simulink model "motor_pendulum_system"  (R2020b)
settings: Solver=VariableStepAuto  StartTime=0.0  StopTime=1  MaxStep=1e-3  RelTol=1e-6
model workspace: external: MATLAB File /Users/sam/GitHub/3-Phase-Motor/Matlab/motor_with_new_controller.m (data not in the file)
values from neighbouring files (symbols this model uses):
  B_m = 1e-3    (= 0.001)    [Calculate_Static.m]    (also in closed_form.m; motor_with_new_controller.m)
  J = 1e-4    (= 0.0001)    [Calculate_Static.m]    (also in closed_form.m; motor_with_new_controller.m)
  K = 0.088    [Calculate_Static.m]    (also in closed_form.m; motor_with_new_controller.m)
libraries: cstblocks x2, pid_lib x2
settings Model: Creator=sam  LastModifiedBy=sam
settings ModelReferenceCC: UpdateModelReferenceTargets=Force

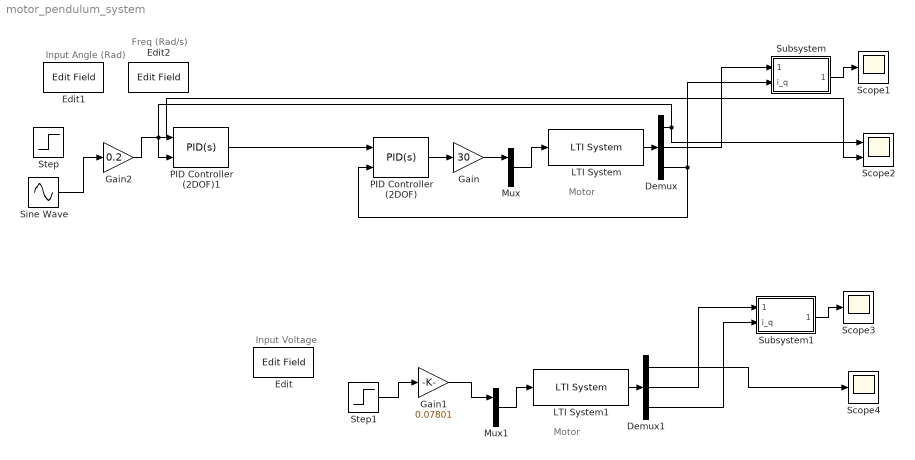
== system motor_pendulum_system ==
  note: Input Voltage
  note: Motor
  note: Motor
  note: Input Angle (Rad)
  note: Freq (Rad/s)
  Demux : Demux  Outputs=3
  Demux1 : Demux  Outputs=3
  Edit : EditField  LabelPosition=Hide  ShowInitialText=on  Alignment=Center
  Edit1 : EditField  LabelPosition=Hide  ShowInitialText=on  Alignment=Center
  Edit2 : EditField  LabelPosition=Hide  ShowInitialText=on  Alignment=Center
  Gain : Gain  Gain=30
  Gain1 : Gain  Gain=0.07801
  Gain2 : Gain  Gain=0.2
  LTI System : cstblocks/LTI System  sys=S  IC=[]
  LTI System1 : cstblocks/LTI System  sys=S  IC=[]
  Mux : Mux  Inputs=3
  Mux1 : Mux  Inputs=3
  PID Controller (2DOF) : pid_lib/PID Controller (2DOF)  Controller=PID  Form=Parallel  TimeDomain=Continuous-time  UseExternalTs=off  SampleTime=-1  IntegratorMethod=Forward Euler  FilterMethod=Forward Euler  ControllerParametersSource=internal  P=.05  I=.005  D=0  UseFilter=on  N=100  b=1  c=1  TunerSelectOption=Transfer Function Based (PID Tuner App)  InitialConditionSource=internal  InitialConditionForIntegrator=0  InitialConditionForFilter=0  DifferentiatorICPrevScaledInput=0  ExternalReset=none  TrackingMode=off  Kt=1  LimitOutput=off  SatLimitsSource=internal  UpperSaturationLimit=inf  LowerSaturationLimit=-inf  LinearizeAsGain=on  AntiWindupMode=none  Kb=1  POutMin=[]  POutMax=[]  IOutMin=[]  IOutMax=[]  DOutMin=[]  DOutMax=[]  NOutMin=[]  NOutMax=[]  bOutMin=[]  bOutMax=[]  cOutMin=[]  cOutMax=[]  SumOutMin=[]  SumOutMax=[]  SaturationOutMin=[]  SaturationOutMax=[]  PParamMin=[]  PParamMax=[]  IParamMin=[]  IParamMax=[]  DParamMin=[]  DParamMax=[]  NParamMin=[]  NParamMax=[]  bParamMin=[]  bParamMax=[]  cParamMin=[]  cParamMax=[]  KbParamMin=[]  KbParamMax=[]  KtParamMin=[]  KtParamMax=[]  KbOutMin=[]  KbOutMax=[]  KtOutMin=[]  KtOutMax=[]  IntegratorOutMin=[]  IntegratorOutMax=[]  FilterOutMin=[]  FilterOutMax=[]  SumI1OutMin=[]  SumI1OutMax=[]  SumI2OutMin=[]  SumI2OutMax=[]  SumI3OutMin=[]  SumI3OutMax=[]  SumI4OutMin=[]  SumI4OutMax=[]  SumDOutMin=[]  SumDOutMax=[]  Sum1OutMin=[]  Sum1OutMax=[]  Sum2OutMin=[]  Sum2OutMax=[]  Sum3OutMin=[]  Sum3OutMax=[]  DifferentiatorOutMin=[]  DifferentiatorOutMax=[]  FilterDiffOutCoefMin=[]  FilterDiffOutCoefMax=[]  ReciprocalOutMin=[]  ReciprocalOutMax=[]  SumDenOutMin=[]  SumDenOutMax=[]  SumNumOutMin=[]  SumNumOutMax=[]  DivideOutMin=[]  DivideOutMax=[]  UdiffTsProdOutMin=[]  UdiffTsProdOutMax=[]  NTsProdOutMin=[]  NTsProdOutMax=[]  UintegralTsProdOutMin=[]  UintegralTsProdOutMax=[]  UngainTsProdOutMin=[]  UngainTsProdOutMax=[]  IntegratorContinuousStateAttributes=''  IntegratorStateMustResolveToSignalObject=off  IntegratorRTWStateStorageClass=Auto  FilterContinuousStateAttributes=''  FilterStateMustResolveToSignalObject=off  FilterRTWStateStorageClass=Auto  ParallelPVariant=InternalParameters  IdealPVariant=Disabled  IVariant=InternalParameters  DVariant=InternalParameters  bVariant=InternalParameters  cVariant=InternalParameters  IntegratorVariant=Continuous  SatVariant=Disabled  AWVariant=Passthrough  PCopyVariant=Disabled  TRVariant=Disabled  FdbkBlocksVariant=Forward  IdealPFdbkVariant=Disabled  SatFdbkVariant=Disabled  DerivativeFilterVariant=ContFilter  NVariant=InternalParameters  NCopyVariant=Disabled  FilterICVariant=InternalICsFilter  IntegratorICVariant=InternalICs  ExternalResetVariant=Disabled  TRSumVariant=Passthrough  SumFdbkVariant=Disabled  SumVariant=Sum_PID  TsampFilterVariant=InternalTs  TsampNgainVariant=Passthrough  TsampIntegralVariant=Passthrough  ExternalSaturationOutDataTypeStr=Inherit: Same as second input
      settings: SourceProductBaseCode=SL
  PID Controller (2DOF)1 : pid_lib/PID Controller (2DOF)  Controller=PID  Form=Parallel  TimeDomain=Continuous-time  UseExternalTs=off  SampleTime=-1  IntegratorMethod=Forward Euler  FilterMethod=Forward Euler  ControllerParametersSource=internal  P=250  I=20  D=5  UseFilter=on  N=100  b=1  c=1  TunerSelectOption=Transfer Function Based (PID Tuner App)  InitialConditionSource=internal  InitialConditionForIntegrator=0  InitialConditionForFilter=0  DifferentiatorICPrevScaledInput=0  ExternalReset=none  TrackingMode=off  Kt=1  LimitOutput=off  SatLimitsSource=internal  UpperSaturationLimit=inf  LowerSaturationLimit=-inf  LinearizeAsGain=on  AntiWindupMode=none  Kb=1  POutMin=[]  POutMax=[]  IOutMin=[]  IOutMax=[]  DOutMin=[]  DOutMax=[]  NOutMin=[]  NOutMax=[]  bOutMin=[]  bOutMax=[]  cOutMin=[]  cOutMax=[]  SumOutMin=[]  SumOutMax=[]  SaturationOutMin=[]  SaturationOutMax=[]  PParamMin=[]  PParamMax=[]  IParamMin=[]  IParamMax=[]  DParamMin=[]  DParamMax=[]  NParamMin=[]  NParamMax=[]  bParamMin=[]  bParamMax=[]  cParamMin=[]  cParamMax=[]  KbParamMin=[]  KbParamMax=[]  KtParamMin=[]  KtParamMax=[]  KbOutMin=[]  KbOutMax=[]  KtOutMin=[]  KtOutMax=[]  IntegratorOutMin=[]  IntegratorOutMax=[]  FilterOutMin=[]  FilterOutMax=[]  SumI1OutMin=[]  SumI1OutMax=[]  SumI2OutMin=[]  SumI2OutMax=[]  SumI3OutMin=[]  SumI3OutMax=[]  SumI4OutMin=[]  SumI4OutMax=[]  SumDOutMin=[]  SumDOutMax=[]  Sum1OutMin=[]  Sum1OutMax=[]  Sum2OutMin=[]  Sum2OutMax=[]  Sum3OutMin=[]  Sum3OutMax=[]  DifferentiatorOutMin=[]  DifferentiatorOutMax=[]  FilterDiffOutCoefMin=[]  FilterDiffOutCoefMax=[]  ReciprocalOutMin=[]  ReciprocalOutMax=[]  SumDenOutMin=[]  SumDenOutMax=[]  SumNumOutMin=[]  SumNumOutMax=[]  DivideOutMin=[]  DivideOutMax=[]  UdiffTsProdOutMin=[]  UdiffTsProdOutMax=[]  NTsProdOutMin=[]  NTsProdOutMax=[]  UintegralTsProdOutMin=[]  UintegralTsProdOutMax=[]  UngainTsProdOutMin=[]  UngainTsProdOutMax=[]  IntegratorContinuousStateAttributes=''  IntegratorStateMustResolveToSignalObject=off  IntegratorRTWStateStorageClass=Auto  FilterContinuousStateAttributes=''  FilterStateMustResolveToSignalObject=off  FilterRTWStateStorageClass=Auto  ParallelPVariant=InternalParameters  IdealPVariant=Disabled  IVariant=InternalParameters  DVariant=InternalParameters  bVariant=InternalParameters  cVariant=InternalParameters  IntegratorVariant=Continuous  SatVariant=Disabled  AWVariant=Passthrough  PCopyVariant=Disabled  TRVariant=Disabled  FdbkBlocksVariant=Forward  IdealPFdbkVariant=Disabled  SatFdbkVariant=Disabled  DerivativeFilterVariant=ContFilter  NVariant=InternalParameters  NCopyVariant=Disabled  FilterICVariant=InternalICsFilter  IntegratorICVariant=InternalICs  ExternalResetVariant=Disabled  TRSumVariant=Passthrough  SumFdbkVariant=Disabled  SumVariant=Sum_PID  TsampFilterVariant=InternalTs  TsampNgainVariant=Passthrough  TsampIntegralVariant=Passthrough  ExternalSaturationOutDataTypeStr=Inherit: Same as second input
      settings: SourceProductBaseCode=SL
  Scope1 : Scope
  Scope2 : Scope  NumInputPorts=2
  Scope3 : Scope
  Scope4 : Scope
  Sine Wave : Sin  Frequency=125.6637061  SampleTime=0
  Step : Step  Time=0  SampleTime=0
  Step1 : Step  Time=0  SampleTime=0
  Subsystem : Subsystem
  Subsystem1 : Subsystem
  wires:
  LTI System/1 -> Demux/1
  PID Controller (2DOF)/1 -> Gain/1
  Gain/1 -> Mux/1
  Mux/1 -> LTI System/1
  PID Controller (2DOF)1/1 -> PID Controller (2DOF)/1
  Subsystem/1(Out1) -> Scope1/1
  LTI System1/1 -> Demux1/1
  Subsystem1/1(Out1) -> Scope3/1
  Mux1/1 -> LTI System1/1
  Step1/1 -> Gain1/1
  Gain2/1 -> Scope2/2, PID Controller (2DOF)1/1
  Demux1/1 -> Scope4/1
  Demux1/2 -> Subsystem1/1(Theta_dot)
  Demux1/3 -> Subsystem1/2(i_q)
  Gain1/1 -> Mux1/1
  Demux/1 -> PID Controller (2DOF)1/2, Scope2/1
  Demux/3 -> PID Controller (2DOF)/2, Subsystem/2(i_q)
  Demux/2 -> Subsystem/1(Theta_dot)
  Sine Wave/1 -> Gain2/1

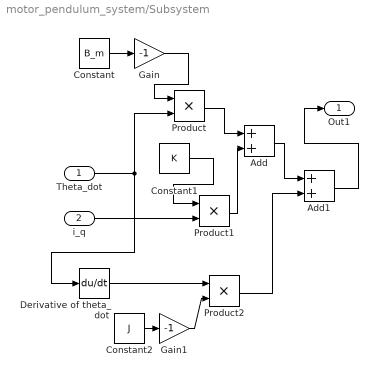
== system motor_pendulum_system/Subsystem ==
  Theta_dot : Inport
  i_q : Inport  Port=2
  Add : Sum
  Add1 : Sum
  Constant : Constant  Value=B_m
  Constant1 : Constant  Value=K
  Constant2 : Constant  Value=J
  Derivative of theta_dot : Derivative
  Gain : Gain  Gain=-1
  Gain1 : Gain  Gain=-1
  Product : Product
  Product1 : Product
  Product2 : Product
  Out1 : Outport
  wires:
  Theta_dot/1 -> Derivative of theta_dot/1, Product/2
  Constant/1 -> Gain/1
  Gain/1 -> Product/1
  Constant1/1 -> Product1/1
  i_q/1 -> Product1/2
  Product/1 -> Add/1
  Product1/1 -> Add/2
  Add/1 -> Add1/1
  Derivative of theta_dot/1 -> Product2/1
  Product2/1 -> Add1/2
  Add1/1 -> Out1/1
  Constant2/1 -> Gain1/1
  Gain1/1 -> Product2/2

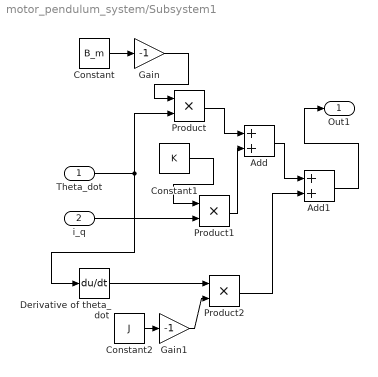
== system motor_pendulum_system/Subsystem1 ==
  Theta_dot : Inport
  i_q : Inport  Port=2
  Add : Sum
  Add1 : Sum
  Constant : Constant  Value=B_m
  Constant1 : Constant  Value=K
  Constant2 : Constant  Value=J
  Derivative of theta_dot : Derivative
  Gain : Gain  Gain=-1
  Gain1 : Gain  Gain=-1
  Product : Product
  Product1 : Product
  Product2 : Product
  Out1 : Outport
  wires:
  Theta_dot/1 -> Derivative of theta_dot/1, Product/2
  Constant/1 -> Gain/1
  Gain/1 -> Product/1
  Constant1/1 -> Product1/1
  i_q/1 -> Product1/2
  Product/1 -> Add/1
  Product1/1 -> Add/2
  Add/1 -> Add1/1
  Derivative of theta_dot/1 -> Product2/1
  Product2/1 -> Add1/2
  Add1/1 -> Out1/1
  Constant2/1 -> Gain1/1
  Gain1/1 -> Product2/2
